simulink model "quad2_jump"  (R2015b)
settings: Solver=FixedStepAuto  StartTime=0.0  StopTime=10  FixedStep=1e-4  MinStep=1e-4  RelTol=1e-2  AbsTol=1e-6
InitFcn:
  | init_quad;
StartFcn:
  | init_quad;
undefined symbols (not defined in the file or in its folder): body, ctrl, planner, sigbuilder_block, X, Y, Z
libraries: nesl_utility x61, sm_lib x41, simulink x4, Contact_Forces_Lib x4, Parts_Lib x4
(part 1 of 3)
settings Model: Creator=Administrator  LastModifiedBy=Administrator
settings SolverCC: MaxConsecutiveMinStep=5  ZeroCrossAlgorithm=Adaptive
settings DebuggingCC: ReadBeforeWriteMsg=DisableAll  WriteAfterWriteMsg=DisableAll  WriteAfterReadMsg=DisableAll  MultiTaskDSMMsg=none
settings DiagnosticsConfigSet: SimMechanicsUnconnectedFramePorts=none  SimMechanicsUnconnectedGeometryPorts=none  SimMechanicsRedundantBlock=none  SimMechanicsRigidlyBoundBlock=none

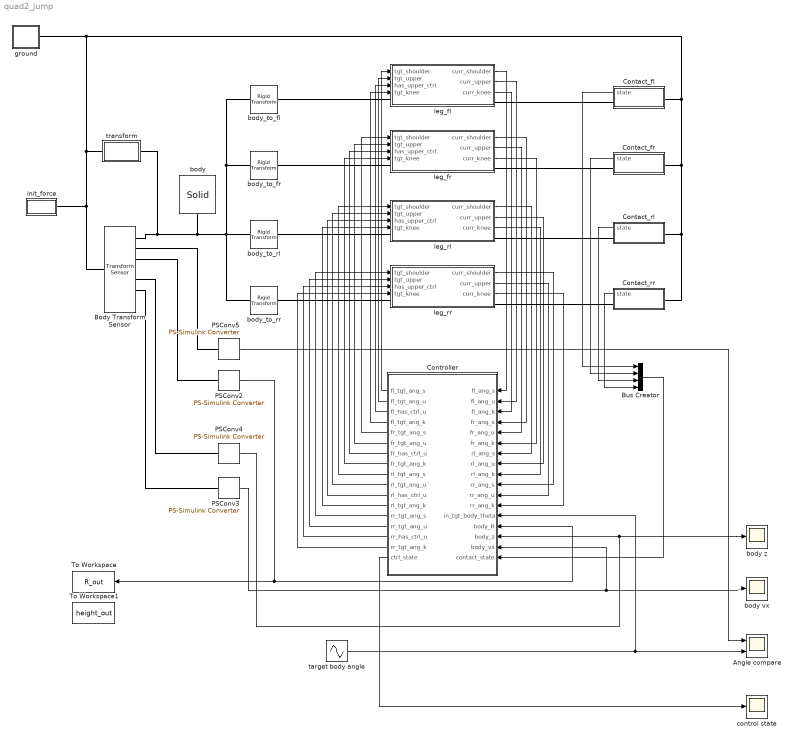
== system quad2_jump ==
  "Angle compare " : Scope  NumInputPorts=2
  Body Transform Sensor : sm_lib/Frames and Transforms/Transform Sensor  MeasurementFrame=World  SenseAngle=on  SenseAxis=off  SenseAngle1=off  SenseAngle2=off  SenseAngle3=off  SenseQ=off  SenseR=on  SenseOmegaX=off  SenseOmegaY=off  SenseOmegaZ=off  SenseOmega1=off  SenseOmega2=off  SenseOmega3=off  SenseQDot=off  SenseRDot=off  SenseAlphaX=off  SenseAlphaY=off  SenseAlphaZ=off  SenseAlpha1=off  SenseAlpha2=off  SenseAlpha3=off  SenseQDDot=off  SenseRDDot=off  SenseX=on  SenseY=off  SenseZ=on  SenseRad=off  SenseAzim=off  SenseDist=off  SenseInc=off  SenseXDot=on  SenseYDot=off  SenseZDot=on  SenseRadDot=off  SenseAzimDot=off  SenseDistDot=off  SenseIncDot=off  SenseXDDot=off  SenseYDDot=off  SenseZDDot=off  SenseRadDDot=off  SenseAzimDDot=off  SenseDistDDot=off  SenseIncDDot=off  BlockFunction=simmechanics.library.frames_transforms.transform_sensor
  Bus Creator : BusCreator  Inputs=4
  Contact_fl : Subsystem
  Contact_fr : Subsystem
  Contact_rl : Subsystem
  Contact_rr : Subsystem
  Controller : MATLAB Function  TreatAsAtomicUnit=on
  PSConv{2..5} (4 alike) : nesl_utility/PS-Simulink Converter  PhysicalDomain=network_engine_domain  SubClassName=ps_output  LeftPortType=input  RightPortType=output  PseudoPeriodic=off  Frequencies=[]  Unit=1  AffineConversion=off
  To Workspace : ToWorkspace  VariableName=R_out  SaveFormat=Structure With Time  SampleTime=-1
  To Workspace1 : ToWorkspace  VariableName=height_out  SaveFormat=Structure With Time  SampleTime=-1
  body : sm_lib/Body Elements/Solid  InertiaType=CalculateFromGeometry  Mass=8.6  MassUnits=kg  CenterOfMass=[0 0 0]  CenterOfMassUnits=m  MomentsOfInertia=[1 1 1]  MomentsOfInertiaUnits=kg*m^2  ProductsOfInertia=[0 0 0]  ProductsOfInertiaUnits=kg*m^2  DensityBased=on  Density=200  DensityUnits=kg/(m^3)  DoExposeReferenceFrame=on  SerializedFrames=<Frames><Frame><Id>Frame2</Id><Value><Name>force</Name><Origin><Source>GeometricFeature</Source><FeatureName>-x surface</FeatureName></Origin><PrimaryAxis><DefinedDirection>+Z</DefinedDirection><Source>ReferenceFrame</Source><SourceDirection>+Z</SourceDirection><FeatureName></FeatureName></PrimaryAxis><SecondaryAxis><DefinedDirection>+X</DefinedDirection><Source>ReferenceFrame</Source><SourceDirection>+X</SourceDirection><FeatureName></FeatureName></SecondaryAxis></Value></Frame></Frames>  GraphicType=FromGeometry  MarkerShape=Sphere  MarkerSize=10  GraphicVisPropType=SimpleVisualProperties  GraphicDiffuseColor=[1.0 0.0 0.2]  GraphicSpecularColor=[0.5 0.5 0.5 1.0]  GraphicAmbientColor=[0.15 0.15 0.15 1.0]  GraphicEmissiveColor=[0.0 0.0 0.0 1.0]  GraphicShininess=75  GraphicOpacity=1.0  GeometryShape=Brick  RectangleSize=[1 1]  RectangleSizeUnits=m  BrickDimensions=[0.6 0.3 0.15]  BrickDimensionUnits=m  CylinderRadius=1  CylinderRadiusUnits=m  CylinderLength=1  CylinderLengthUnits=m  SphereRadius=1  SphereRadiusUnits=m  EllipsoidRadii=[1 1 1]  EllipsoidRadiiUnits=m  ExtrusionCrossSection=[1 1; -1 1; -1 -1; 1 -1]  ExtrusionCrossSectionUnits=m  ExtrusionLength=1  ExtrusionLengthUnits=m  PolygonNumSides=3  PolygonOuterRadius=1  PolygonOuterRadiusUnits=m  ExtGeomFileType=STL  ExtGeomFileUnits=m  RevolutionCrossSection=[1 1; 1 -1; 2 -1; 2 1]  RevolutionCrossSectionUnits=m  RevolutionExtent=Full  RevolutionAngle=180  RevolutionAngleUnits=deg  BlockFunction=simmechanics.library.body_elements.solid
  "body vx " : Scope
  body z : Scope
  body_to_fl : sm_lib/Frames and Transforms/Rigid Transform  TranslationMethod=Cartesian  TranslationLengthUnit=m  TranslationStandardAxis=+Z  TranslationStandardOffset=0  TranslationCartesianOffset=[0.2 0.15+0.035 0]  TranslationROffset=0  TranslationROffsetUnits=m  TranslationZOffset=0  TranslationZOffsetUnits=m  TranslationThetaOffset=0  TranslationThetaOffsetUnits=deg  RotationMethod=AlignedAxes  RotationAngleUnits=deg  RotationStandardAxis=+Z  RotationAngle=0.0  RotationArbitraryAxis=[0 0 1]  FollAlignAxisA=+Z  BaseAlignAxisA=+X  FollAlignAxisB=+X  BaseAlignAxisB=-Z  RotationSequenceAxes=FollowerAxes  RotationSequence=XYX  RotationSequenceAngles=[0 0 0]  RotationSequenceAnglesUnits=deg  RotationMatrix=[1 0 0; 0 1 0; 0 0 1]  BlockFunction=simmechanics.library.frames_transforms.rigid_transform
  body_to_fr : sm_lib/Frames and Transforms/Rigid Transform  TranslationMethod=Cartesian  TranslationLengthUnit=m  TranslationStandardAxis=+Z  TranslationStandardOffset=0  TranslationCartesianOffset=[0.2 -0.15-0.035 0]  TranslationROffset=0  TranslationROffsetUnits=m  TranslationZOffset=0  TranslationZOffsetUnits=m  TranslationThetaOffset=0  TranslationThetaOffsetUnits=deg  RotationMethod=AlignedAxes  RotationAngleUnits=deg  RotationStandardAxis=+Z  RotationAngle=0.0  RotationArbitraryAxis=[0 0 1]  FollAlignAxisA=+Z  BaseAlignAxisA=+X  FollAlignAxisB=+X  BaseAlignAxisB=-Z  RotationSequenceAxes=FollowerAxes  RotationSequence=XYX  RotationSequenceAngles=[0 0 0]  RotationSequenceAnglesUnits=deg  RotationMatrix=[1 0 0; 0 1 0; 0 0 1]  BlockFunction=simmechanics.library.frames_transforms.rigid_transform
  body_to_rl : sm_lib/Frames and Transforms/Rigid Transform  TranslationMethod=Cartesian  TranslationLengthUnit=m  TranslationStandardAxis=+Z  TranslationStandardOffset=0  TranslationCartesianOffset=[-0.2 0.15+0.035 0]  TranslationROffset=0  TranslationROffsetUnits=m  TranslationZOffset=0  TranslationZOffsetUnits=m  TranslationThetaOffset=0  TranslationThetaOffsetUnits=deg  RotationMethod=AlignedAxes  RotationAngleUnits=deg  RotationStandardAxis=+Z  RotationAngle=0.0  RotationArbitraryAxis=[0 0 1]  FollAlignAxisA=+Z  BaseAlignAxisA=+X  FollAlignAxisB=+X  BaseAlignAxisB=-Z  RotationSequenceAxes=FollowerAxes  RotationSequence=XYX  RotationSequenceAngles=[0 0 0]  RotationSequenceAnglesUnits=deg  RotationMatrix=[1 0 0; 0 1 0; 0 0 1]  BlockFunction=simmechanics.library.frames_transforms.rigid_transform
  body_to_rr : sm_lib/Frames and Transforms/Rigid Transform  TranslationMethod=Cartesian  TranslationLengthUnit=m  TranslationStandardAxis=+Z  TranslationStandardOffset=0  TranslationCartesianOffset=[-0.2 -0.15-0.035 0]  TranslationROffset=0  TranslationROffsetUnits=m  TranslationZOffset=0  TranslationZOffsetUnits=m  TranslationThetaOffset=0  TranslationThetaOffsetUnits=deg  RotationMethod=AlignedAxes  RotationAngleUnits=deg  RotationStandardAxis=+Z  RotationAngle=0.0  RotationArbitraryAxis=[0 0 1]  FollAlignAxisA=+Z  BaseAlignAxisA=+X  FollAlignAxisB=+X  BaseAlignAxisB=-Z  RotationSequenceAxes=FollowerAxes  RotationSequence=XYX  RotationSequenceAngles=[0 0 0]  RotationSequenceAnglesUnits=deg  RotationMatrix=[1 0 0; 0 1 0; 0 0 1]  BlockFunction=simmechanics.library.frames_transforms.rigid_transform
  "control state " : Scope
  ground : Subsystem
  init_force : Subsystem
  leg_fl : Subsystem
  leg_fr : Subsystem
  leg_rl : Subsystem
  leg_rr : Subsystem
  "target body angle " : Sin  Amplitude=15*pi/180  Frequency=3  SampleTime=0
  transform : Subsystem
  wires:
  PSConv2/1 -> Controller/14(body_R), To Workspace/1
  leg_fl/1(curr_shoulder) -> Controller/1(fl_ang_s)
  leg_fl/2("curr_upper ") -> Controller/2(fl_ang_u)
  leg_fl/3(curr_knee) -> Controller/3(fl_ang_k)
  leg_fr/1(curr_shoulder) -> Controller/4(fr_ang_s)
  leg_fr/2("curr_upper ") -> Controller/5(fr_ang_u)
  leg_fr/3(curr_knee) -> Controller/6(fr_ang_k)
  leg_rl/1(curr_shoulder) -> Controller/7(rl_ang_s)
  leg_rl/2("curr_upper ") -> Controller/8(rl_ang_u)
  leg_rl/3(curr_knee) -> Controller/9(rl_ang_k)
  leg_rr/1(curr_shoulder) -> Controller/10(rr_ang_s)
  leg_rr/2("curr_upper ") -> Controller/11(rr_ang_u)
  leg_rr/3(curr_knee) -> Controller/12(rr_ang_k)
  PSConv4/1 -> body z/1, Controller/15(body_z)
  PSConv3/1 -> Controller/16(body_vx), "body vx "/1
  Controller/1(fl_tgt_ang_s) -> leg_fl/1(tgt_shoulder)
  Controller/2(fl_tgt_ang_u) -> leg_fl/2(tgt_upper)
  Controller/3(fl_has_ctrl_u) -> leg_fl/3(has_upper_ctrl)
  Controller/4(fl_tgt_ang_k) -> leg_fl/4(tgt_knee)
  Controller/5(fr_tgt_ang_s) -> leg_fr/1(tgt_shoulder)
  Controller/6(fr_tgt_ang_u) -> leg_fr/2(tgt_upper)
  Controller/7(fr_has_ctrl_u) -> leg_fr/3(has_upper_ctrl)
  Controller/8(fr_tgt_ang_k) -> leg_fr/4(tgt_knee)
  Controller/9(rl_tgt_ang_s) -> leg_rl/1(tgt_shoulder)
  Controller/10(rl_tgt_ang_u) -> leg_rl/2(tgt_upper)
  Controller/11(rl_has_ctrl_u) -> leg_rl/3(has_upper_ctrl)
  Controller/12(rl_tgt_ang_k) -> leg_rl/4(tgt_knee)
  Controller/13(rr_tgt_ang_s) -> leg_rr/1(tgt_shoulder)
  Controller/14(rr_tgt_ang_u) -> leg_rr/2(tgt_upper)
  Controller/15(rr_has_ctrl_u) -> leg_rr/3(has_upper_ctrl)
  Controller/16(rr_tgt_ang_k) -> leg_rr/4(tgt_knee)
  Bus Creator/1 -> Controller/17(contact_state)
  Contact_fl/1(state) -> Bus Creator/1
  Contact_fr/1(state) -> Bus Creator/2
  Contact_rl/1(state) -> Bus Creator/3
  Contact_rr/1(state) -> Bus Creator/4
  "target body angle "/1 -> Controller/13(in_tgt_body_theta), "Angle compare "/2
  PSConv5/1 -> "Angle compare "/1
  Controller/17(ctrl_state) -> "control state "/1
  connections:
  ground/RConn1 -- Contact_rr/LConn1 -- Contact_rl/LConn1 -- Contact_fr/LConn1 -- Contact_fl/LConn1 -- transform/RConn1 -- Body Transform Sensor/LConn1 -- init_force/LConn1
  transform/LConn1 -- body_to_fr/LConn1 -- body_to_fl/LConn1 -- body_to_rl/LConn1 -- body_to_rr/LConn1 -- body/RConn1 -- Body Transform Sensor/RConn1
  leg_rl/RConn1 -- Contact_rl/RConn1
  body_to_rl/RConn1 -- leg_rl/LConn1
  leg_rr/RConn1 -- Contact_rr/RConn1
  body_to_rr/RConn1 -- leg_rr/LConn1
  leg_fr/RConn1 -- Contact_fr/RConn1
  Contact_fl/RConn1 -- leg_fl/RConn1
  body_to_fl/RConn1 -- leg_fl/LConn1
  body_to_fr/RConn1 -- leg_fr/LConn1
  Body Transform Sensor/RConn3 -- PSConv2/LConn1
  PSConv4/LConn1 -- Body Transform Sensor/RConn5
  PSConv3/LConn1 -- Body Transform Sensor/RConn6
  PSConv5/LConn1 -- Body Transform Sensor/RConn2

== system quad2_jump/Contact_fl ==
  note: state 4 166.31ms
  note: 这是一个蛋疼的处理，因为地面现在厚度是0.4，为了和碰撞的block要求匹配，所以碰撞是相对于这个地面的中心来算的。而检测高度的时候就要把这个厚度减掉
      | 但是Transform sensor要检测的是球和地面的高度差
  Bus Selector : BusSelector  OutputSignals=Normal Force,Frame Sep,Friction Force
  Compare To Constant : simulink/Logic and Bit Operations/Compare To Constant  relop=<=  const=planner.touch_down_height  OutDataTypeStr=uint8
  PSConv4 : nesl_utility/PS-Simulink Converter  PhysicalDomain=network_engine_domain  SubClassName=ps_output  LeftPortType=input  RightPortType=output  PseudoPeriodic=off  Frequencies=[]  Unit=1  AffineConversion=off
  Sphere to Plane Force1 : Contact_Forces_Lib/3D/Sphere to Plane Force  sphere_rad=body.foot_radius  plane_lenx=12  plane_leny=12  plane_depth=0.2  force_law=Linear  k_contact=ground.stiff  b_contact=ground.damp  pen_full_damp_F=1e-4  pen_exponent=1  custom_param_1=1  custom_param_2=1  friction_law=Stick-Slip Continuous  mu_kinetic=0.7  mu_static=0.7  v_thr=0.001
  State Scope : Scope
  Terminator : Terminator
  Transform Sensor : sm_lib/Frames and Transforms/Transform Sensor  MeasurementFrame=World  SenseAngle=off  SenseAxis=off  SenseAngle1=off  SenseAngle2=off  SenseAngle3=off  SenseQ=off  SenseR=off  SenseOmegaX=off  SenseOmegaY=off  SenseOmegaZ=off  SenseOmega1=off  SenseOmega2=off  SenseOmega3=off  SenseQDot=off  SenseRDot=off  SenseAlphaX=off  SenseAlphaY=off  SenseAlphaZ=off  SenseAlpha1=off  SenseAlpha2=off  SenseAlpha3=off  SenseQDDot=off  SenseRDDot=off  SenseX=off  SenseY=off  SenseZ=on  SenseRad=off  SenseAzim=off  SenseDist=off  SenseInc=off  SenseXDot=off  SenseYDot=off  SenseZDot=off  SenseRadDot=off  SenseAzimDot=off  SenseDistDot=off  SenseIncDot=off  SenseXDDot=off  SenseYDDot=off  SenseZDDot=off  SenseRadDDot=off  SenseAzimDDot=off  SenseDistDDot=off  SenseIncDDot=off  BlockFunction=simmechanics.library.frames_transforms.transform_sensor
  ZScope : Scope
  force : Scope  NumInputPorts=2
  PlanB : PMIOPort  Port=1  Side=Left
  SphF : PMIOPort  Port=2  Side=Right
  state : Outport
  wires:
  Sphere to Plane Force1/1 -> Bus Selector/1
  Bus Selector/1 -> force/1  "<Normal Force>"
  PSConv4/1 -> Compare To Constant/1, ZScope/1
  Compare To Constant/1 -> state/1, State Scope/1
  Bus Selector/3 -> force/2  "<Friction Force>"
  Bus Selector/2 -> Terminator/1  "<Frame Sep>"
  connections:
  Sphere to Plane Force1/LConn1 -- Transform Sensor/RConn1 -- SphF/RConn1
  Sphere to Plane Force1/RConn1 -- Transform Sensor/LConn1 -- PlanB/RConn1
  PSConv4/LConn1 -- Transform Sensor/RConn2

== system quad2_jump/Contact_fr ==
  note: state 4 166.31ms
  note: 这是一个蛋疼的处理，因为地面现在厚度是0.4，为了和碰撞的block要求匹配，所以碰撞是相对于这个地面的中心来算的。而检测高度的时候就要把这个厚度减掉
      | 但是Transform sensor要检测的是球和地面的高度差
  Bus Selector : BusSelector  OutputSignals=Normal Force,Frame Sep,Friction Force
  Compare To Constant : simulink/Logic and Bit Operations/Compare To Constant  relop=<=  const=planner.touch_down_height  OutDataTypeStr=uint8
  PSConv4 : nesl_utility/PS-Simulink Converter  PhysicalDomain=network_engine_domain  SubClassName=ps_output  LeftPortType=input  RightPortType=output  PseudoPeriodic=off  Frequencies=[]  Unit=1  AffineConversion=off
  Sphere to Plane Force1 : Contact_Forces_Lib/3D/Sphere to Plane Force  sphere_rad=body.foot_radius  plane_lenx=12  plane_leny=12  plane_depth=0.2  force_law=Linear  k_contact=ground.stiff  b_contact=ground.damp  pen_full_damp_F=1e-4  pen_exponent=1  custom_param_1=1  custom_param_2=1  friction_law=Stick-Slip Continuous  mu_kinetic=0.7  mu_static=0.7  v_thr=0.001
  State Scope : Scope
  Terminator : Terminator
  Transform Sensor : sm_lib/Frames and Transforms/Transform Sensor  MeasurementFrame=World  SenseAngle=off  SenseAxis=off  SenseAngle1=off  SenseAngle2=off  SenseAngle3=off  SenseQ=off  SenseR=off  SenseOmegaX=off  SenseOmegaY=off  SenseOmegaZ=off  SenseOmega1=off  SenseOmega2=off  SenseOmega3=off  SenseQDot=off  SenseRDot=off  SenseAlphaX=off  SenseAlphaY=off  SenseAlphaZ=off  SenseAlpha1=off  SenseAlpha2=off  SenseAlpha3=off  SenseQDDot=off  SenseRDDot=off  SenseX=off  SenseY=off  SenseZ=on  SenseRad=off  SenseAzim=off  SenseDist=off  SenseInc=off  SenseXDot=off  SenseYDot=off  SenseZDot=off  SenseRadDot=off  SenseAzimDot=off  SenseDistDot=off  SenseIncDot=off  SenseXDDot=off  SenseYDDot=off  SenseZDDot=off  SenseRadDDot=off  SenseAzimDDot=off  SenseDistDDot=off  SenseIncDDot=off  BlockFunction=simmechanics.library.frames_transforms.transform_sensor
  ZScope : Scope
  force : Scope  NumInputPorts=2
  PlanB : PMIOPort  Port=1  Side=Left
  SphF : PMIOPort  Port=2  Side=Right
  state : Outport
  wires:
  Sphere to Plane Force1/1 -> Bus Selector/1
  Bus Selector/1 -> force/1  "<Normal Force>"
  PSConv4/1 -> Compare To Constant/1, ZScope/1
  Compare To Constant/1 -> state/1, State Scope/1
  Bus Selector/3 -> force/2  "<Friction Force>"
  Bus Selector/2 -> Terminator/1  "<Frame Sep>"
  connections:
  Sphere to Plane Force1/LConn1 -- Transform Sensor/RConn1 -- SphF/RConn1
  Sphere to Plane Force1/RConn1 -- Transform Sensor/LConn1 -- PlanB/RConn1
  PSConv4/LConn1 -- Transform Sensor/RConn2

== system quad2_jump/Contact_rl ==
  note: 这是一个蛋疼的处理，因为地面现在厚度是0.4，为了和碰撞的block要求匹配，所以碰撞是相对于这个地面的中心来算的。而检测高度的时候就要把这个厚度减掉
      | 但是Transform sensor要检测的是球和地面的高度差
  Bus Selector : BusSelector  OutputSignals=Normal Force,Frame Sep,Friction Force
  Compare To Constant : simulink/Logic and Bit Operations/Compare To Constant  relop=<=  const=planner.touch_down_height  OutDataTypeStr=uint8
  PSConv4 : nesl_utility/PS-Simulink Converter  PhysicalDomain=network_engine_domain  SubClassName=ps_output  LeftPortType=input  RightPortType=output  PseudoPeriodic=off  Frequencies=[]  Unit=1  AffineConversion=off
  Sphere to Plane Force1 : Contact_Forces_Lib/3D/Sphere to Plane Force  sphere_rad=body.foot_radius  plane_lenx=12  plane_leny=12  plane_depth=0.2  force_law=Linear  k_contact=ground.stiff  b_contact=ground.damp  pen_full_damp_F=1e-4  pen_exponent=1  custom_param_1=1  custom_param_2=1  friction_law=Stick-Slip Continuous  mu_kinetic=0.7  mu_static=0.7  v_thr=0.001
  State Scope : Scope
  Terminator : Terminator
  Transform Sensor : sm_lib/Frames and Transforms/Transform Sensor  MeasurementFrame=World  SenseAngle=off  SenseAxis=off  SenseAngle1=off  SenseAngle2=off  SenseAngle3=off  SenseQ=off  SenseR=off  SenseOmegaX=off  SenseOmegaY=off  SenseOmegaZ=off  SenseOmega1=off  SenseOmega2=off  SenseOmega3=off  SenseQDot=off  SenseRDot=off  SenseAlphaX=off  SenseAlphaY=off  SenseAlphaZ=off  SenseAlpha1=off  SenseAlpha2=off  SenseAlpha3=off  SenseQDDot=off  SenseRDDot=off  SenseX=off  SenseY=off  SenseZ=on  SenseRad=off  SenseAzim=off  SenseDist=off  SenseInc=off  SenseXDot=off  SenseYDot=off  SenseZDot=off  SenseRadDot=off  SenseAzimDot=off  SenseDistDot=off  SenseIncDot=off  SenseXDDot=off  SenseYDDot=off  SenseZDDot=off  SenseRadDDot=off  SenseAzimDDot=off  SenseDistDDot=off  SenseIncDDot=off  BlockFunction=simmechanics.library.frames_transforms.transform_sensor
  ZScope : Scope
  force : Scope  NumInputPorts=2
  PlanB : PMIOPort  Port=1  Side=Left
  SphF : PMIOPort  Port=2  Side=Right
  state : Outport
  wires:
  Sphere to Plane Force1/1 -> Bus Selector/1
  Bus Selector/1 -> force/1  "<Normal Force>"
  PSConv4/1 -> Compare To Constant/1, ZScope/1
  Compare To Constant/1 -> state/1, State Scope/1
  Bus Selector/3 -> force/2  "<Friction Force>"
  Bus Selector/2 -> Terminator/1  "<Frame Sep>"
  connections:
  Sphere to Plane Force1/LConn1 -- Transform Sensor/RConn1 -- SphF/RConn1
  Sphere to Plane Force1/RConn1 -- Transform Sensor/LConn1 -- PlanB/RConn1
  PSConv4/LConn1 -- Transform Sensor/RConn2

== system quad2_jump/Contact_rr ==
  note: state 4 166.31ms
  note: 这是一个蛋疼的处理，因为地面现在厚度是0.4，为了和碰撞的block要求匹配，所以碰撞是相对于这个地面的中心来算的。而检测高度的时候就要把这个厚度减掉
      | 但是Transform sensor要检测的是球和地面的高度差
  Bus Selector : BusSelector  OutputSignals=Normal Force,Frame Sep,Friction Force
  Compare To Constant : simulink/Logic and Bit Operations/Compare To Constant  relop=<=  const=planner.touch_down_height  OutDataTypeStr=uint8
  PSConv4 : nesl_utility/PS-Simulink Converter  PhysicalDomain=network_engine_domain  SubClassName=ps_output  LeftPortType=input  RightPortType=output  PseudoPeriodic=off  Frequencies=[]  Unit=1  AffineConversion=off
  Sphere to Plane Force1 : Contact_Forces_Lib/3D/Sphere to Plane Force  sphere_rad=body.foot_radius  plane_lenx=12  plane_leny=12  plane_depth=0.2  force_law=Linear  k_contact=ground.stiff  b_contact=ground.damp  pen_full_damp_F=1e-4  pen_exponent=1  custom_param_1=1  custom_param_2=1  friction_law=Stick-Slip Continuous  mu_kinetic=0.7  mu_static=0.7  v_thr=0.001
  State Scope : Scope
  Terminator : Terminator
  Transform Sensor : sm_lib/Frames and Transforms/Transform Sensor  MeasurementFrame=World  SenseAngle=off  SenseAxis=off  SenseAngle1=off  SenseAngle2=off  SenseAngle3=off  SenseQ=off  SenseR=off  SenseOmegaX=off  SenseOmegaY=off  SenseOmegaZ=off  SenseOmega1=off  SenseOmega2=off  SenseOmega3=off  SenseQDot=off  SenseRDot=off  SenseAlphaX=off  SenseAlphaY=off  SenseAlphaZ=off  SenseAlpha1=off  SenseAlpha2=off  SenseAlpha3=off  SenseQDDot=off  SenseRDDot=off  SenseX=off  SenseY=off  SenseZ=on  SenseRad=off  SenseAzim=off  SenseDist=off  SenseInc=off  SenseXDot=off  SenseYDot=off  SenseZDot=off  SenseRadDot=off  SenseAzimDot=off  SenseDistDot=off  SenseIncDot=off  SenseXDDot=off  SenseYDDot=off  SenseZDDot=off  SenseRadDDot=off  SenseAzimDDot=off  SenseDistDDot=off  SenseIncDDot=off  BlockFunction=simmechanics.library.frames_transforms.transform_sensor
  ZScope : Scope
  force : Scope  NumInputPorts=2
  PlanB : PMIOPort  Port=1  Side=Left
  SphF : PMIOPort  Port=2  Side=Right
  state : Outport
  wires:
  Sphere to Plane Force1/1 -> Bus Selector/1
  Bus Selector/1 -> force/1  "<Normal Force>"
  PSConv4/1 -> Compare To Constant/1, ZScope/1
  Compare To Constant/1 -> state/1, State Scope/1
  Bus Selector/3 -> force/2  "<Friction Force>"
  Bus Selector/2 -> Terminator/1  "<Frame Sep>"
  connections:
  Sphere to Plane Force1/LConn1 -- Transform Sensor/RConn1 -- SphF/RConn1
  Sphere to Plane Force1/RConn1 -- Transform Sensor/LConn1 -- PlanB/RConn1
  PSConv4/LConn1 -- Transform Sensor/RConn2

== system quad2_jump/ground ==
  Mechanism Configuration : sm_lib/Utilities/Mechanism Configuration  UniformGravity=Constant  GravityVector=[0 0 -9.80665]  GravityUnits=m/s^2  LinearizationDelta=0.001  BlockFunction=simmechanics.library.utilities.mechanism_configuration
  Solver Configuration : nesl_utility/Solver Configuration  PhysicalDomain=network_engine_domain  SubClassName=solver  LeftPortType=input  RightPortType=generic  Accelerate=off  Tones=[]  Harmonics=[]  SimulateNoise=off  Profile=off  UseLocalSampling=off  EnableSwitchedLinearOptims=on  FrequencyDomain=off  UseCCode=off  RelTol=0.001  AbsTol=1e-06  MinStep=1e-09  ToWorkspace=off  RevertToSquareIcSolve=off  NumHomotopyIterations=100  PhasorMode=off  PhasorModeNumHarmonics=1  DoDC=off  ResidualTolerance=1e-09  UseLocalSolver=off  LocalSolverChoice=NE_BACKWARD_EULER_ADVANCER  LocalSolverSampleTime=0.001  DoFixedCost=off  MaxNonlinIter=3  MaxModeIter=2  LinearAlgebra=Sparse  DelaysMemoryBudget=1024  AutomaticFiltering=on  FilteringTimeConstant=0.001
  World Frame : sm_lib/Frames and Transforms/World Frame  BlockFunction=simmechanics.library.frames_transforms.world_frame
  ground : sm_lib/Body Elements/Solid  InertiaType=CalculateFromGeometry  Mass=1  MassUnits=kg  CenterOfMass=[0 0 0]  CenterOfMassUnits=m  MomentsOfInertia=[1 1 1]  MomentsOfInertiaUnits=kg*m^2  ProductsOfInertia=[0 0 0]  ProductsOfInertiaUnits=kg*m^2  DensityBased=on  Density=1000  DensityUnits=kg/(m^3)  DoExposeReferenceFrame=on  SerializedFrames=<Frames/>  GraphicType=FromGeometry  MarkerShape=Sphere  MarkerSize=10  GraphicVisPropType=SimpleVisualProperties  GraphicDiffuseColor=[0.6 1.0 0.8]  GraphicSpecularColor=[0.5 0.5 0.5 1.0]  GraphicAmbientColor=[0.15 0.15 0.15 1.0]  GraphicEmissiveColor=[0.0 0.0 0.0 1.0]  GraphicShininess=75  GraphicOpacity=1.0  GeometryShape=Brick  RectangleSize=[1 1]  RectangleSizeUnits=m  BrickDimensions=[12 12 0.4]  BrickDimensionUnits=m  CylinderRadius=1  CylinderRadiusUnits=m  CylinderLength=1  CylinderLengthUnits=m  SphereRadius=1  SphereRadiusUnits=m  EllipsoidRadii=[1 1 1]  EllipsoidRadiiUnits=m  ExtrusionCrossSection=[1 1; -1 1; -1 -1; 1 -1]  ExtrusionCrossSectionUnits=m  ExtrusionLength=1  ExtrusionLengthUnits=m  PolygonNumSides=3  PolygonOuterRadius=1  PolygonOuterRadiusUnits=m  ExtGeomFileType=STL  ExtGeomFileUnits=m  RevolutionCrossSection=[1 1; 1 -1; 2 -1; 2 1]  RevolutionCrossSectionUnits=m  RevolutionExtent=Full  RevolutionAngle=180  RevolutionAngleUnits=deg  BlockFunction=simmechanics.library.body_elements.solid
  port1 : PMIOPort  Port=1  Side=Right
  connections:
  Solver Configuration/RConn1 -- World Frame/RConn1 -- port1/RConn1 -- ground/RConn1 -- Mechanism Configuration/RConn1

== system quad2_jump/init_force ==
  External Force and Torque1 : sm_lib/Forces and Torques/External Force and Torque  ForceResolutionFrame=AttachedFrame  EnableForceX=on  EnableForceY=off  EnableForceZ=off  EnableForce=off  TorqueResolutionFrame=AttachedFrame  EnableTorqueX=on  EnableTorqueY=off  EnableTorqueZ=off  EnableTorque=off  BlockFunction=simmechanics.library.forces_torques.external_force_torque
  Signal Builder : Subsystem  Tag=STV Subsys  LoadFcn=sigbuilder_block('load');  StartFcn=sigbuilder_block('start');  StopFcn=sigbuilder_block('stop');  ClipboardFcn=sigbuilder_block('clipboard');  mask(Sigbuilder block){}
      mask help: Simulink:masks:SigbuilderBlock_MD
      mask init:
      | if ~strcmp(get_param(bdroot(gcbh),'SimulationStatus'),'stopped') tuvar = sigbuilder_block('maskInit'); end
      settings: CopyFcn=sigbuilder_block('copy');  DeleteFcn=sigbuilder_block('delete');  ModelCloseFcn=sigbuilder_block('modelClose');  PreSaveFcn=sigbuilder_block('preSave');  PauseFcn=sigbuilder_block('pause');  ContinueFcn=sigbuilder_block('continue');  NameChangeFcn=sigbuilder_block('namechange');  OpenFcn=sigbuilder_block('open',[437.25 108.75 550.5 358.5 ]);  CloseFcn=sigbuilder_block('close');
      mask Display: plot(0, 0, 100, 100,[2, 2, 32, 32, 2], [68, 8, 8, 68, 68],[32, 2], [38, 38], [32, 19, 2],[53, 60, 44], [32, 17, 17, 2],[16, 16, 31, 31]);txt = getActiveGroup(gcbh);text(2, 100, txt,'verticalAlignment', 'top');
  Simulink-PS Converter1 : nesl_utility/Simulink-PS Converter  PhysicalDomain=network_engine_domain  SubClassName=ps_input  LeftPortType=input  RightPortType=output  PseudoPeriodic=off  Frequencies=[]  NoiseDistribution=none  NoiseParameters=[]  Unit=1  AffineConversion=off  InputFiltering=off  SimscapeFilterOrder=1  InputFilterTimeConstant=0.001  UdotUserProvided=1
  Conn1 : PMIOPort  Port=1  Side=Left
  wires:
  Signal Builder/1(Signal 1) -> Simulink-PS Converter1/1
  connections:
  External Force and Torque1/RConn1 -- Conn1/RConn1
  Simulink-PS Converter1/RConn1 -- External Force and Torque1/LConn2 -- External Force and Torque1/LConn1

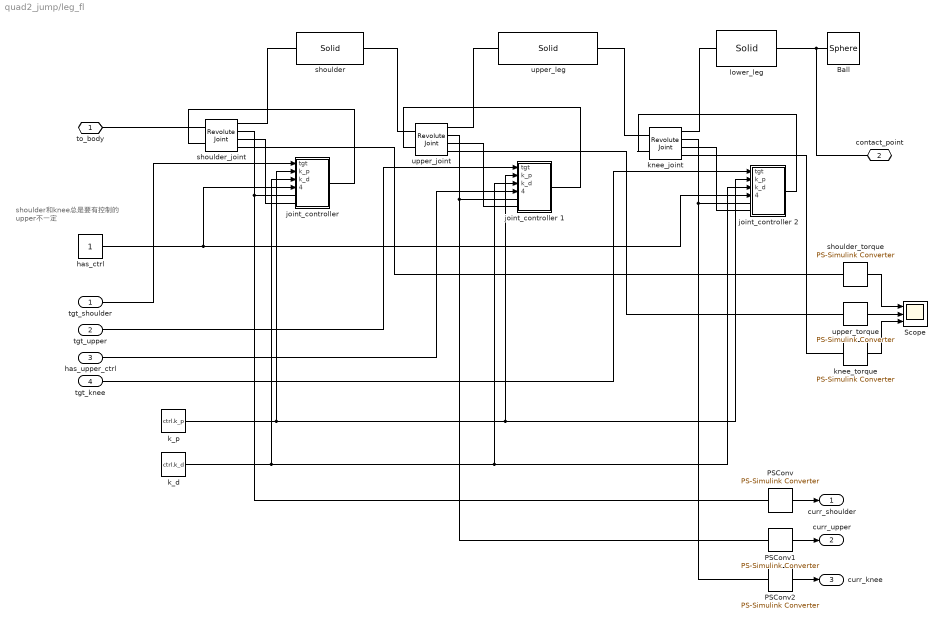
== system quad2_jump/leg_fl ==
  note: shoulder和knee总是要有控制的
      | upper不一定
  tgt_shoulder : Inport
  tgt_upper : Inport  Port=2
  has_upper_ctrl : Inport  Port=3
  tgt_knee : Inport  Port=4
  Ball : Parts_Lib/Sphere  Tag=CustomStyle  sph_radius=0.035  sph_density=1000  sph_color=red  sph_opacity=1  mark_type=Rings on center planes  arc_width=[40 50]  arc_angle=60  ring_width=5  ring_irad=0.95  mark_color=axes  mark_opacity=1  ring_opacity=0  arc_opacity=0
  PSConv : nesl_utility/PS-Simulink Converter  PhysicalDomain=network_engine_domain  SubClassName=ps_output  LeftPortType=input  RightPortType=output  PseudoPeriodic=off  Frequencies=[]  Unit=1  AffineConversion=off
  PSConv1 : nesl_utility/PS-Simulink Converter  PhysicalDomain=network_engine_domain  SubClassName=ps_output  LeftPortType=input  RightPortType=output  PseudoPeriodic=off  Frequencies=[]  Unit=1  AffineConversion=off
  PSConv2 : nesl_utility/PS-Simulink Converter  PhysicalDomain=network_engine_domain  SubClassName=ps_output  LeftPortType=input  RightPortType=output  PseudoPeriodic=off  Frequencies=[]  Unit=1  AffineConversion=off
  Scope : Scope  NumInputPorts=3
  "has_ctrl " : Constant
  "joint_controller " : Subsystem
  joint_controller 1 : Subsystem
  joint_controller 2 : Subsystem
  k_d : Constant  Value=ctrl.k_d
  k_p : Constant  Value=ctrl.k_p
  knee_joint : sm_lib/Joints/Revolute Joint  SenseConstraintForce=off  SenseConstraintForceX=off  SenseConstraintForceY=off  SenseConstraintForceZ=off  SenseConstraintTorque=off  SenseConstraintTorqueX=off  SenseConstraintTorqueY=off  SenseConstraintTorqueZ=off  SenseTotalForce=off  SenseTotalForceX=off  SenseTotalForceY=off  SenseTotalForceZ=off  SenseTotalTorque=off  SenseTotalTorqueX=off  SenseTotalTorqueY=off  SenseTotalTorqueZ=off  CompositeWrenchDir=FollowerOnBase  CompositeWrenchFrame=BaseFrame  EquilibriumPosition=0  EquilibriumPositionUnits=deg  SpringStiffness=0  SpringStiffnessUnits=N*m/rad  DampingCoefficient=0  DampingCoefficientUnits=N*m/(deg/s)  TorqueActuationMode=InputTorque  MotionActuationMode=ComputedMotion  SensePosition=on  SenseVelocity=on  SenseAcceleration=off  SenseTorqueForce=on  PositionTargetSpecify=off  PositionTargetPriority=High  PositionTargetValue=0  PositionTargetValueUnits=deg  VelocityTargetSpecify=off  VelocityTargetPriority=High  VelocityTargetValue=0  VelocityTargetValueUnits=deg/s  BlockFunction=simmechanics.library.joints.revolute_joint
  knee_torque : nesl_utility/PS-Simulink Converter  PhysicalDomain=network_engine_domain  SubClassName=ps_output  LeftPortType=input  RightPortType=output  PseudoPeriodic=off  Frequencies=[]  Unit=1  AffineConversion=off
  lower_leg : sm_lib/Body Elements/Solid  InertiaType=CalculateFromGeometry  Mass=1  MassUnits=kg  CenterOfMass=[0 0 0]  CenterOfMassUnits=m  MomentsOfInertia=[1 1 1]  MomentsOfInertiaUnits=kg*m^2  ProductsOfInertia=[0 0 0]  ProductsOfInertiaUnits=kg*m^2  DensityBased=on  Density=660  DensityUnits=kg/(m^3)  DoExposeReferenceFrame=off  SerializedFrames=<Frames><Frame><Id>Frame1</Id><Value><Name>joint_knee</Name><Origin><Source>GeometricFeature</Source><FeatureName>+z surface</FeatureName></Origin><PrimaryAxis><DefinedDirection>+Z</DefinedDirection><Source>ReferenceFrame</Source><SourceDirection>+Y</SourceDirection><FeatureName></FeatureName></PrimaryAxis><SecondaryAxis><DefinedDirection>+X</DefinedDirection><Source>ReferenceFrame</Source><SourceDirection>+X</SourceDirection><FeatureName></FeatureName></SecondaryAxis></Value></Frame><Frame><Id>Frame2</Id><Value><Name>td_F</Name><Origin><Source>GeometricFeature</Source><FeatureName>-z surface</FeatureName></Origin><PrimaryAxis><DefinedDirection>+Z</DefinedDirection><Source>ReferenceFrame</Source><SourceDirection>+Z</SourceDirection><FeatureName></FeatureName></PrimaryAxis><SecondaryAxis><DefinedDirection>+X</DefinedDirection><Source>ReferenceFrame</Source><SourceDirection>+X</SourceDirection><FeatureName></FeatureName></SecondaryAxis></Value></Frame></Frames>  GraphicType=FromGeometry  MarkerShape=Sphere  MarkerSize=10  GraphicVisPropType=SimpleVisualProperties  GraphicDiffuseColor=[0.6 0.2 1.0]  GraphicSpecularColor=[0.5 0.5 0.5 1.0]  GraphicAmbientColor=[0.15 0.15 0.15 1.0]  GraphicEmissiveColor=[0.0 0.0 0.0 1.0]  GraphicShininess=75  GraphicOpacity=1.0  GeometryShape=Brick  RectangleSize=[1 1]  RectangleSizeUnits=m  BrickDimensions=[0.04 0.04 0.2]  BrickDimensionUnits=m  CylinderRadius=1  CylinderRadiusUnits=m  CylinderLength=1  CylinderLengthUnits=m  SphereRadius=1  SphereRadiusUnits=m  EllipsoidRadii=[1 1 1]  EllipsoidRadiiUnits=m  ExtrusionCrossSection=[1 1; -1 1; -1 -1; 1 -1]  ExtrusionCrossSectionUnits=m  ExtrusionLength=1  ExtrusionLengthUnits=m  PolygonNumSides=3  PolygonOuterRadius=1  PolygonOuterRadiusUnits=m  ExtGeomFileType=STL  ExtGeomFileUnits=m  RevolutionCrossSection=[1 1; 1 -1; 2 -1; 2 1]  RevolutionCrossSectionUnits=m  RevolutionExtent=Full  RevolutionAngle=180  RevolutionAngleUnits=deg  BlockFunction=simmechanics.library.body_elements.solid
  shoulder : sm_lib/Body Elements/Solid  InertiaType=CalculateFromGeometry  Mass=1  MassUnits=kg  CenterOfMass=[0 0 0]  CenterOfMassUnits=m  MomentsOfInertia=[1 1 1]  MomentsOfInertiaUnits=kg*m^2  ProductsOfInertia=[0 0 0]  ProductsOfInertiaUnits=kg*m^2  DensityBased=on  Density=660  DensityUnits=kg/(m^3)  DoExposeReferenceFrame=off  SerializedFrames=<Frames><Frame><Id>Frame1</Id><Value><Name>to_body</Name><Origin><Source>CenterOfMassFrame</Source><FeatureName></FeatureName></Origin><PrimaryAxis><DefinedDirection>+Z</DefinedDirection><Source>ReferenceFrame</Source><SourceDirection>+X</SourceDirection><FeatureName></FeatureName></PrimaryAxis><SecondaryAxis><DefinedDirection>+X</DefinedDirection><Source>ReferenceFrame</Source><SourceDirection>-Z</SourceDirection><FeatureName></FeatureName></SecondaryAxis></Value></Frame><Frame><Id>Frame2</Id><Value><Name>to_leg</Name><Origin><Source>ReferenceFrame</Source><FeatureName></FeatureName></Origin><PrimaryAxis><DefinedDirection>+Z</DefinedDirection><Source>ReferenceFrame</Source><SourceDirection>+Y</SourceDirection><FeatureName></FeatureName></PrimaryAxis><SecondaryAxis><DefinedDirection>+X</DefinedDirection><Source>ReferenceFrame</Source><SourceDirection>+X</SourceDirection><FeatureName></FeatureName></SecondaryAxis></Value></Frame></Frames>  GraphicType=FromGeometry  MarkerShape=Sphere  MarkerSize=10  GraphicVisPropType=SimpleVisualProperties  GraphicDiffuseColor=[0.4 1.0 0.0]  GraphicSpecularColor=[0.5 0.5 0.5 1.0]  GraphicAmbientColor=[0.15 0.15 0.15 1.0]  GraphicEmissiveColor=[0.0 0.0 0.0 1.0]  GraphicShininess=75  GraphicOpacity=1.0  GeometryShape=Brick  RectangleSize=[1 1]  RectangleSizeUnits=m  BrickDimensions=[0.07 0.07 0.07]  BrickDimensionUnits=m  CylinderRadius=1  CylinderRadiusUnits=m  CylinderLength=1  CylinderLengthUnits=m  SphereRadius=1  SphereRadiusUnits=m  EllipsoidRadii=[1 1 1]  EllipsoidRadiiUnits=m  ExtrusionCrossSection=[1 1; -1 1; -1 -1; 1 -1]  ExtrusionCrossSectionUnits=m  ExtrusionLength=1  ExtrusionLengthUnits=m  PolygonNumSides=3  PolygonOuterRadius=1  PolygonOuterRadiusUnits=m  ExtGeomFileType=STL  ExtGeomFileUnits=m  RevolutionCrossSection=[1 1; 1 -1; 2 -1; 2 1]  RevolutionCrossSectionUnits=m  RevolutionExtent=Full  RevolutionAngle=180  RevolutionAngleUnits=deg  BlockFunction=simmechanics.library.body_elements.solid
  shoulder_joint : sm_lib/Joints/Revolute Joint  SenseConstraintForce=off  SenseConstraintForceX=off  SenseConstraintForceY=off  SenseConstraintForceZ=off  SenseConstraintTorque=off  SenseConstraintTorqueX=off  SenseConstraintTorqueY=off  SenseConstraintTorqueZ=off  SenseTotalForce=off  SenseTotalForceX=off  SenseTotalForceY=off  SenseTotalForceZ=off  SenseTotalTorque=off  SenseTotalTorqueX=off  SenseTotalTorqueY=off  SenseTotalTorqueZ=off  CompositeWrenchDir=FollowerOnBase  CompositeWrenchFrame=BaseFrame  EquilibriumPosition=0  EquilibriumPositionUnits=deg  SpringStiffness=0  SpringStiffnessUnits=N*m/deg  DampingCoefficient=0  DampingCoefficientUnits=N*m/(deg/s)  TorqueActuationMode=InputTorque  MotionActuationMode=ComputedMotion  SensePosition=on  SenseVelocity=on  SenseAcceleration=off  SenseTorqueForce=on  PositionTargetSpecify=off  PositionTargetPriority=High  PositionTargetValue=0  PositionTargetValueUnits=deg  VelocityTargetSpecify=off  VelocityTargetPriority=High  VelocityTargetValue=0  VelocityTargetValueUnits=deg/s  BlockFunction=simmechanics.library.joints.revolute_joint
  shoulder_torque : nesl_utility/PS-Simulink Converter  PhysicalDomain=network_engine_domain  SubClassName=ps_output  LeftPortType=input  RightPortType=output  PseudoPeriodic=off  Frequencies=[]  Unit=1  AffineConversion=off
  upper_joint : sm_lib/Joints/Revolute Joint  SenseConstraintForce=off  SenseConstraintForceX=off  SenseConstraintForceY=off  SenseConstraintForceZ=off  SenseConstraintTorque=off  SenseConstraintTorqueX=off  SenseConstraintTorqueY=off  SenseConstraintTorqueZ=off  SenseTotalForce=off  SenseTotalForceX=off  SenseTotalForceY=off  SenseTotalForceZ=off  SenseTotalTorque=off  SenseTotalTorqueX=off  SenseTotalTorqueY=off  SenseTotalTorqueZ=off  CompositeWrenchDir=FollowerOnBase  CompositeWrenchFrame=BaseFrame  EquilibriumPosition=0  EquilibriumPositionUnits=deg  SpringStiffness=0  SpringStiffnessUnits=N*m/deg  DampingCoefficient=0  DampingCoefficientUnits=N*m/(deg/s)  TorqueActuationMode=InputTorque  MotionActuationMode=ComputedMotion  SensePosition=on  SenseVelocity=on  SenseAcceleration=off  SenseTorqueForce=on  PositionTargetSpecify=off  PositionTargetPriority=High  PositionTargetValue=0  PositionTargetValueUnits=deg  VelocityTargetSpecify=off  VelocityTargetPriority=High  VelocityTargetValue=0  VelocityTargetValueUnits=deg/s  BlockFunction=simmechanics.library.joints.revolute_joint
  upper_leg : sm_lib/Body Elements/Solid  InertiaType=CalculateFromGeometry  Mass=1  MassUnits=kg  CenterOfMass=[0 0 0]  CenterOfMassUnits=m  MomentsOfInertia=[1 1 1]  MomentsOfInertiaUnits=kg*m^2  ProductsOfInertia=[0 0 0]  ProductsOfInertiaUnits=kg*m^2  DensityBased=on  Density=660  DensityUnits=kg/(m^3)  DoExposeReferenceFrame=off  SerializedFrames=<Frames><Frame><Id>Frame1</Id><Value><Name>to_shoulder</Name><Origin><Source>GeometricFeature</Source><FeatureName>+z surface</FeatureName></Origin><PrimaryAxis><DefinedDirection>+Z</DefinedDirection><Source>ReferenceFrame</Source><SourceDirection>+Y</SourceDirection><FeatureName></FeatureName></PrimaryAxis><SecondaryAxis><DefinedDirection>+X</DefinedDirection><Source>ReferenceFrame</Source><SourceDirection>+X</SourceDirection><FeatureName></FeatureName></SecondaryAxis></Value></Frame><Frame><Id>Frame2</Id><Value><Name>joint_knee</Name><Origin><Source>GeometricFeature</Source><FeatureName>-z surface</FeatureName></Origin><PrimaryAxis><DefinedDirection>+Z</DefinedDirection><Source>ReferenceFrame</Source><SourceDirection>+Y</SourceDirection><FeatureName></FeatureName></PrimaryAxis><SecondaryAxis><DefinedDirection>+X</DefinedDirection><Source>ReferenceFrame</Source><SourceDirection>+X</SourceDirection><FeatureName></FeatureName></SecondaryAxis></Value></Frame></Frames>  GraphicType=FromGeometry  MarkerShape=Sphere  MarkerSize=10  GraphicVisPropType=SimpleVisualProperties  GraphicDiffuseColor=[0.8 0.0 0.8]  GraphicSpecularColor=[0.5 0.5 0.5 1.0]  GraphicAmbientColor=[0.15 0.15 0.15 1.0]  GraphicEmissiveColor=[0.0 0.0 0.0 1.0]  GraphicShininess=75  GraphicOpacity=1.0  GeometryShape=Brick  RectangleSize=[1 1]  RectangleSizeUnits=m  BrickDimensions=[0.04 0.04 0.2]  BrickDimensionUnits=m  CylinderRadius=1  CylinderRadiusUnits=m  CylinderLength=1  CylinderLengthUnits=m  SphereRadius=1  SphereRadiusUnits=m  EllipsoidRadii=[1 1 1]  EllipsoidRadiiUnits=m  ExtrusionCrossSection=[1 1; -1 1; -1 -1; 1 -1]  ExtrusionCrossSectionUnits=m  ExtrusionLength=1  ExtrusionLengthUnits=m  PolygonNumSides=3  PolygonOuterRadius=1  PolygonOuterRadiusUnits=m  ExtGeomFileType=STL  ExtGeomFileUnits=m  RevolutionCrossSection=[1 1; 1 -1; 2 -1; 2 1]  RevolutionCrossSectionUnits=m  RevolutionExtent=Full  RevolutionAngle=180  RevolutionAngleUnits=deg  BlockFunction=simmechanics.library.body_elements.solid
  upper_torque : nesl_utility/PS-Simulink Converter  PhysicalDomain=network_engine_domain  SubClassName=ps_output  LeftPortType=input  RightPortType=output  PseudoPeriodic=off  Frequencies=[]  Unit=1  AffineConversion=off
  to_body : PMIOPort  Port=1  Side=Left
  contact_point : PMIOPort  Port=2  Side=Right
  curr_shoulder : Outport
  "curr_upper " : Outport  Port=2
  curr_knee : Outport  Port=3
  wires:
  tgt_shoulder/1 -> "joint_controller "/1(tgt)
  tgt_upper/1 -> joint_controller 1/1(tgt)
  k_p/1 -> "joint_controller "/2(k_p), joint_controller 2/2(k_p), joint_controller 1/2(k_p)
  k_d/1 -> "joint_controller "/3(k_d), joint_controller 2/3(k_d), joint_controller 1/3(k_d)
  tgt_knee/1 -> joint_controller 2/1(tgt)
  "has_ctrl "/1 -> joint_controller 2/4(has_ctrl), "joint_controller "/4(has_ctrl)
  has_upper_ctrl/1 -> joint_controller 1/4(has_ctrl)
  PSConv/1 -> curr_shoulder/1
  PSConv1/1 -> "curr_upper "/1
  PSConv2/1 -> curr_knee/1
  shoulder_torque/1 -> Scope/1
  upper_torque/1 -> Scope/2
  knee_torque/1 -> Scope/3
  connections:
  contact_point/RConn1 -- Ball/LConn1 -- lower_leg/RConn1
  upper_joint/RConn1 -- upper_leg/LConn1
  knee_joint/LConn1 -- upper_leg/RConn1
  knee_joint/RConn1 -- lower_leg/LConn1
  to_body/RConn1 -- shoulder_joint/LConn1
  shoulder/RConn1 -- upper_joint/LConn1
  shoulder_joint/RConn1 -- shoulder/LConn1
  shoulder_joint/RConn2 -- PSConv/LConn1 -- "joint_controller "/LConn1
  "joint_controller "/RConn1 -- shoulder_joint/LConn2
  shoulder_joint/RConn3 -- "joint_controller "/LConn2
  upper_joint/RConn2 -- PSConv1/LConn1 -- joint_controller 1/LConn1
  joint_controller 1/RConn1 -- upper_joint/LConn2
  upper_joint/RConn3 -- joint_controller 1/LConn2
  knee_joint/RConn2 -- PSConv2/LConn1 -- joint_controller 2/LConn1
  joint_controller 2/LConn2 -- knee_joint/RConn3
  knee_joint/LConn2 -- joint_controller 2/RConn1
  shoulder_torque/LConn1 -- shoulder_joint/RConn4
  upper_torque/LConn1 -- upper_joint/RConn4
  knee_torque/LConn1 -- knee_joint/RConn4
